simulink model "exp11_1"  (R2020a)
settings: Solver=VariableStepAuto  StartTime=0.0  StopTime=10.0  RelTol=1e-3
settings Model: Creator=zengw  LastModifiedBy=zengw

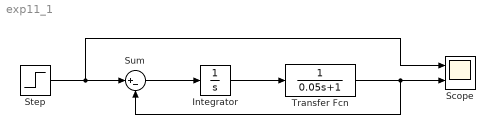
== system exp11_1 ==
  Integrator : Integrator
  Scope : Scope  NumInputPorts=2
  Step : Step  Time=0  SampleTime=0
  Sum : Sum  Inputs=|+-
  Transfer Fcn : TransferFcn  Denominator=[0.05 1]
  wires:
  Integrator/1 -> Transfer Fcn/1
  Transfer Fcn/1 -> Sum/2, Scope/2
  Sum/1 -> Integrator/1
  Step/1 -> Sum/1, Scope/1
